simulink model "ADMIRE"  (R2021b)
settings: Solver=ode4  StartTime=0.0  StopTime=100  FixedStep=1e-2  RelTol=1e-3
undefined symbols (not defined in the file or in its folder): admireDB, Earth, WGS84
libraries: simulink_extras x112, simulink x27, aerolibutil x4, dspsigops x4, aerolibfltsims x3, sharedtransform x2, aerolibtransform2 x2, aerolibatmos2 x1, matrix_library x1, sharedutil x1, aerolibanimutils x1, vrlib x1
(part 3 of 15)

== system ADMIRE/Aircraft/Aerodynamics/YawMomentCoefficient/MachRegion2 ==
  note: 0.4 < Mach < 0.5
  AeroIn_Bus : Inport
  Bus Creator : BusCreator  Inputs=3
  Cymbasic : Subsystem
  Cymbcai : Subsystem
  Cymbde : Subsystem
  Cymbdle : Subsystem
  Cymbdn : Subsystem
  Cymbeta : Subsystem
  Cymbetad : Subsystem
  Cymblg : Subsystem
  Cymdai : Subsystem
  Cymdaib : Subsystem
  Cymday : Subsystem
  Cymdayb : Subsystem
  Cymdna : Subsystem
  Cymdr : Subsystem
  Cymp : Subsystem
  Cympbeta : Subsystem
  Cymr : Subsystem
  Cymrbeta : Subsystem
  Sum : Sum  Inputs=18
  eoeff : Subsystem
  Cymtot : Outport
  wires:
  Cympbeta/1(Cympbeta) -> Sum/16  "Cympbeta"
  eoeff/2(eieff) -> Bus Creator/3  "eieff"
  Cymdaib/1(Cymdaib) -> Sum/10  "Cymdaib"
  Cymbdle/1(Cymbdle) -> Sum/5  "Cymbdle"
  Cymdr/1(Cymdr) -> Sum/8  "Cymdr"
  Cymr/1(Cymr) -> Sum/17  "Cymr"
  Cymdayb/1(Cymdayb) -> Sum/12  "Cymdayb"
  Cymdai/1(Cymdai) -> Sum/9  "Cymdai"
  Cymrbeta/1(Cymrbeta) -> Sum/18  "Cymrbeta"
  Bus Creator/1 -> Cympbeta/1(in_bus), Cymr/1(in_bus), Cymrbeta/1(in_bus), Cymp/1(in_bus), Cymbetad/1(in_bus), Cymdna/1(in_bus), Cymdayb/1(in_bus), Cymday/1(in_bus), Cymdaib/1(in_bus), Cymdai/1(in_bus), Cymdr/1(in_bus), Cymblg/1(in_bus), Cymbcai/1(in_bus), Cymbdle/1(in_bus), Cymbdn/1(in_bus), Cymbde/1(in_bus), Cymbeta/1(in_bus), Cymbasic/1(in_bus)  "in_bus"
  eoeff/1(eoeff) -> Bus Creator/2  "eoeff"
  Cymbasic/1(Cymbasic) -> Sum/1  "Cymbasic"
  Cymblg/1(Cymblg) -> Sum/7  "Cymblg"
  Cymbde/1(Cymbde) -> Sum/3  "Cymbde"
  AeroIn_Bus/1 -> eoeff/1(AeroIn_Bus), Bus Creator/1
  Cymbcai/1(Cymbcai) -> Sum/6  "Cymbcai"
  Cymbeta/1(Cymbeta) -> Sum/2  "Cymbeta"
  Cymbdn/1(Cymbdn) -> Sum/4  "Cymbdn"
  Cymp/1(Cymp) -> Sum/15  "Cymp"
  Cymbetad/1(Cymbetad) -> Sum/14  "Cymbetad"
  Cymday/1(Cymday) -> Sum/11  "Cymday"
  Cymdna/1(Cymdna) -> Sum/13  "Cymdna"
  Sum/1 -> Cymtot/1

== system ADMIRE/Aircraft/Aerodynamics/YawMomentCoefficient/MachRegion3 ==
  note: 0.5 <= Mach <= 1.4
  AeroIn_Bus : Inport
  Bus Creator : BusCreator  Inputs=3
  Cymbasic : Subsystem
  Cymbcai : Subsystem
  Cymbde : Subsystem
  Cymbdle : Subsystem
  Cymbdn : Subsystem
  Cymbeta : Subsystem
  Cymbetad : Subsystem
  Cymblg : Subsystem
  Cymdai : Subsystem
  Cymdaib : Subsystem
  Cymday : Subsystem
  Cymdayb : Subsystem
  Cymdna : Subsystem
  Cymdr : Subsystem
  Cymp : Subsystem
  Cympbeta : Subsystem
  Cymr : Subsystem
  Cymrbeta : Subsystem
  Sum : Sum  Inputs=18
  eoeff : Subsystem
  Cymtot : Outport
  wires:
  Cymbasic/1(Cymbasic) -> Sum/1  "Cymbasic"
  Cymp/1(Cymp) -> Sum/15  "Cymp"
  Cymday/1(Cymday) -> Sum/11  "Cymday"
  AeroIn_Bus/1 -> eoeff/1(AeroIn_Bus), Bus Creator/1
  Cympbeta/1(Cympbeta) -> Sum/16  "Cympbeta"
  Cymbde/1(Cymbde) -> Sum/3  "Cymbde"
  Cymdna/1(Cymdna) -> Sum/13  "Cymdna"
  Cymbdn/1(Cymbdn) -> Sum/4  "Cymbdn"
  Bus Creator/1 -> Cymr/1(in_bus), Cymp/1(in_bus), Cymbetad/1(in_bus), Cymdna/1(in_bus), Cymday/1(in_bus), Cymdai/1(in_bus), Cymdr/1(in_bus), Cymblg/1(in_bus), Cymbcai/1(in_bus), Cymbdle/1(in_bus), Cymbdn/1(in_bus), Cymbde/1(in_bus), Cymbeta/1(in_bus)  "in_bus"
  eoeff/2(eieff) -> Bus Creator/3  "eieff"
  Cymdaib/1(Cymdaib) -> Sum/10  "Cymdaib"
  Cymblg/1(Cymblg) -> Sum/7  "Cymblg"
  eoeff/1(eoeff) -> Bus Creator/2  "eoeff"
  Cymdayb/1(Cymdayb) -> Sum/12  "Cymdayb"
  Cymbdle/1(Cymbdle) -> Sum/5  "Cymbdle"
  Cymdr/1(Cymdr) -> Sum/8  "Cymdr"
  Cymdai/1(Cymdai) -> Sum/9  "Cymdai"
  Cymr/1(Cymr) -> Sum/17  "Cymr"
  Cymbetad/1(Cymbetad) -> Sum/14  "Cymbetad"
  Cymbcai/1(Cymbcai) -> Sum/6  "Cymbcai"
  Cymrbeta/1(Cymrbeta) -> Sum/18  "Cymrbeta"
  Cymbeta/1(Cymbeta) -> Sum/2  "Cymbeta"
  Sum/1 -> Cymtot/1

== system ADMIRE/Aircraft/Aerodynamics/YawMomentCoefficient/MachRegion4 ==
  note: 1.4 < Mach
  AeroIn_Bus : Inport
  Bus Creator : BusCreator  Inputs=3
  Cymbasic : Subsystem
  Cymbcai : Subsystem
  Cymbde : Subsystem
  Cymbdle : Subsystem
  Cymbdn : Subsystem
  Cymbeta : Subsystem
  Cymbetad : Subsystem
  Cymblg : Subsystem
  Cymdai : Subsystem
  Cymdaib : Subsystem
  Cymday : Subsystem
  Cymdayb : Subsystem
  Cymdna : Subsystem
  Cymdr : Subsystem
  Cymp : Subsystem
  Cympbeta : Subsystem
  Cymr : Subsystem
  Cymrbeta : Subsystem
  Sum : Sum  Inputs=18
  eoeff : Subsystem
  Cymtot : Outport
  wires:
  Sum/1 -> Cymtot/1
  Cymbeta/1(Cymbeta) -> Sum/2  "Cymbeta"
  Cymrbeta/1(Cymrbeta) -> Sum/18  "Cymrbeta"
  Cymbcai/1(Cymbcai) -> Sum/6  "Cymbcai"
  Cymbetad/1(Cymbetad) -> Sum/14  "Cymbetad"
  Cymr/1(Cymr) -> Sum/17  "Cymr"
  Cymdai/1(Cymdai) -> Sum/9  "Cymdai"
  Cymdr/1(Cymdr) -> Sum/8  "Cymdr"
  Cymbdle/1(Cymbdle) -> Sum/5  "Cymbdle"
  Cymdayb/1(Cymdayb) -> Sum/12  "Cymdayb"
  eoeff/1(eoeff) -> Bus Creator/2  "eoeff"
  Cymblg/1(Cymblg) -> Sum/7  "Cymblg"
  Cymdaib/1(Cymdaib) -> Sum/10  "Cymdaib"
  eoeff/2(eieff) -> Bus Creator/3  "eieff"
  Bus Creator/1 -> Cymbeta/1(in_bus), Cymbde/1(in_bus), Cymbdn/1(in_bus), Cymbdle/1(in_bus), Cymbcai/1(in_bus), Cymblg/1(in_bus), Cymdr/1(in_bus), Cymdai/1(in_bus), Cymday/1(in_bus), Cymdna/1(in_bus), Cymbetad/1(in_bus), Cymp/1(in_bus), Cymr/1(in_bus)  "in_bus"
  Cymbdn/1(Cymbdn) -> Sum/4  "Cymbdn"
  Cymdna/1(Cymdna) -> Sum/13  "Cymdna"
  Cymbde/1(Cymbde) -> Sum/3  "Cymbde"
  Cympbeta/1(Cympbeta) -> Sum/16  "Cympbeta"
  AeroIn_Bus/1 -> Bus Creator/1, eoeff/1(AeroIn_Bus)
  Cymday/1(Cymday) -> Sum/11  "Cymday"
  Cymp/1(Cymp) -> Sum/15  "Cymp"
  Cymbasic/1(Cymbasic) -> Sum/1  "Cymbasic"

== system ADMIRE/Aircraft/Aerodynamics/YawMomentCoefficient/Subsystem ==
  mach_nd : Inport
  CymtotMR1 : Inport  Port=2
  CymtotMR2 : Inport  Port=3
  CymtotMR3 : Inport  Port=4
  CymtotMR4 : Inport  Port=5
  AND : Logic  IconShape=distinctive  AllPortsSameDT=off  OutDataTypeStr=boolean
  AND1 : Logic  IconShape=distinctive  AllPortsSameDT=off  OutDataTypeStr=boolean
  Compare To Constant1 : simulink/Logic and Bit Operations/Compare To Constant  relop=<=  const=0.4  OutDataTypeStr=boolean
  Compare To Constant2 : simulink/Logic and Bit Operations/Compare To Constant  relop=>  const=0.4  OutDataTypeStr=boolean
  Compare To Constant3 : simulink/Logic and Bit Operations/Compare To Constant  relop=<  const=0.5  OutDataTypeStr=boolean
  Compare To Constant4 : simulink/Logic and Bit Operations/Compare To Constant  relop=<=  const=1.4  OutDataTypeStr=boolean
  Compare To Constant5 : simulink/Logic and Bit Operations/Compare To Constant  relop=>=  const=0.5  OutDataTypeStr=boolean
  Switch : Switch  Criteria=u2 ~= 0
  Switch1 : Switch  Criteria=u2 ~= 0
  Switch2 : Switch  Criteria=u2 ~= 0
  Cymtot : Outport
  wires:
  Compare To Constant5/1 -> AND1/1
  Compare To Constant4/1 -> AND1/2
  AND1/1 -> Switch2/2
  CymtotMR4/1 -> Switch2/3
  CymtotMR3/1 -> Switch2/1
  Switch/1 -> Cymtot/1
  Switch2/1 -> Switch1/3
  CymtotMR2/1 -> Switch1/1
  Switch1/1 -> Switch/3
  CymtotMR1/1 -> Switch/1
  AND/1 -> Switch1/2
  Compare To Constant3/1 -> AND/2
  Compare To Constant2/1 -> AND/1
  Compare To Constant1/1 -> Switch/2
  mach_nd/1 -> Compare To Constant1/1, Compare To Constant3/1, Compare To Constant4/1, Compare To Constant5/1, Compare To Constant2/1

== system ADMIRE/Aircraft/ControlSurfaces/Actuator/Directfeed ==
  In Bus Element : Inport  PortName=actIn  Element=outElevonRCmd_deg
  In Bus Element1 : Inport  PortName=actIn  Element=canardRCmd_deg
  In Bus Element2 : Inport  PortName=actIn  Element=rudderCmd_deg
  In Bus Element3 : Inport  PortName=actIn  Element=thrustCmd_pct
  In Bus Element4 : Inport  PortName=actIn  Element=canardLCmd_deg
  In Bus Element5 : Inport  PortName=actIn  Element=outElevonLCmd_deg
  In Bus Element6 : Inport  PortName=actIn  Element=inElevonLCmd_deg
  In Bus Element7 : Inport  PortName=actIn  Element=inElevonRCmd_deg
  In Bus Element8 : Inport  PortName=actIn  Element=lefCmd_deg
  In Bus Element9 : Inport  PortName=actIn  Element=lgCmd_bool
  Out Bus Element : Outport  PortName=actOut  Element=outElevonR_deg
  Out Bus Element1 : Outport  PortName=actOut  Element=canardR_deg
  Out Bus Element2 : Outport  PortName=actOut  Element=rudder_deg
  Out Bus Element3 : Outport  PortName=actOut  Element=thrust_pct
  Out Bus Element4 : Outport  PortName=actOut  Element=canardL_deg
  Out Bus Element5 : Outport  PortName=actOut  Element=outElevonL_deg
  Out Bus Element6 : Outport  PortName=actOut  Element=inElevonL_deg
  Out Bus Element7 : Outport  PortName=actOut  Element=inElevonR_deg
  Out Bus Element8 : Outport  PortName=actOut  Element=lef_deg
  Out Bus Element9 : Outport  PortName=actOut  Element=lg_bool
  wires:
  In Bus Element/1 -> Out Bus Element/1
  In Bus Element1/1 -> Out Bus Element1/1
  In Bus Element2/1 -> Out Bus Element2/1
  In Bus Element3/1 -> Out Bus Element3/1
  In Bus Element4/1 -> Out Bus Element4/1
  In Bus Element5/1 -> Out Bus Element5/1
  In Bus Element6/1 -> Out Bus Element6/1
  In Bus Element7/1 -> Out Bus Element7/1
  In Bus Element8/1 -> Out Bus Element8/1
  In Bus Element9/1 -> Out Bus Element9/1

== system ADMIRE/Aircraft/ControlSurfaces/Actuator/FirstOrder ==
  In Bus Element : Inport  PortName=actIn  Element=outElevonRCmd_deg
  In Bus Element1 : Inport  PortName=actIn  Element=canardRCmd_deg
  In Bus Element2 : Inport  PortName=actIn  Element=rudderCmd_deg
  In Bus Element3 : Inport  PortName=actIn  Element=thrustCmd_pct
  In Bus Element4 : Inport  PortName=actIn  Element=canardLCmd_deg
  In Bus Element5 : Inport  PortName=actIn  Element=outElevonLCmd_deg
  In Bus Element6 : Inport  PortName=actIn  Element=inElevonLCmd_deg
  In Bus Element7 : Inport  PortName=actIn  Element=inElevonRCmd_deg
  In Bus Element8 : Inport  PortName=actIn  Element=lefCmd_deg
  In Bus Element9 : Inport  PortName=actIn  Element=lgCmd_bool
  canardL : Subsystem
  inElevonL : Subsystem
  inElevonR : Subsystem
  lef : Subsystem
  outCanardR : Subsystem
  outElevonL : Subsystem
  outElevonR : Subsystem
  rudder : Subsystem
  Out Bus Element : Outport  PortName=actOut  Element=outElevonR_deg
  Out Bus Element1 : Outport  PortName=actOut  Element=canardR_deg
  Out Bus Element2 : Outport  PortName=actOut  Element=rudder_deg
  Out Bus Element3 : Outport  PortName=actOut  Element=thrust_pct
  Out Bus Element4 : Outport  PortName=actOut  Element=canardL_deg
  Out Bus Element5 : Outport  PortName=actOut  Element=outElevonL_deg
  Out Bus Element6 : Outport  PortName=actOut  Element=inElevonL_deg
  Out Bus Element7 : Outport  PortName=actOut  Element=inElevonR_deg
  Out Bus Element8 : Outport  PortName=actOut  Element=lef_deg
  Out Bus Element9 : Outport  PortName=actOut  Element=lg_bool
  wires:
  In Bus Element/1 -> outElevonR/1(actIn)
  In Bus Element1/1 -> outCanardR/1(actIn)
  In Bus Element2/1 -> rudder/1(actIn)
  In Bus Element4/1 -> canardL/1(actIn)
  In Bus Element5/1 -> outElevonL/1(actIn)
  In Bus Element6/1 -> inElevonL/1(actIn)
  In Bus Element7/1 -> inElevonR/1(actIn)
  In Bus Element8/1 -> lef/1(actIn)
  outElevonR/1(actOut) -> Out Bus Element/1
  outCanardR/1(actOut) -> Out Bus Element1/1
  In Bus Element9/1 -> Out Bus Element9/1
  lef/1(actOut) -> Out Bus Element8/1
  inElevonR/1(actOut) -> Out Bus Element7/1
  inElevonL/1(actOut) -> Out Bus Element6/1
  outElevonL/1(actOut) -> Out Bus Element5/1
  canardL/1(actOut) -> Out Bus Element4/1
  In Bus Element3/1 -> Out Bus Element3/1
  rudder/1(actOut) -> Out Bus Element2/1

== system ADMIRE/Aircraft/Equtions of Motion/Angular Speeds/Subsystem ==
  In1 : Inport
  Bus Selector : BusSelector  OutputSignals=Aero_Bus.aeroMomentBodyX_N,Aero_Bus.aeroMomentBodyY_N,Aero_Bus.aeroMomentBodyZ_N
  Ground : Ground
  Mux : Mux  Inputs=3
  Mux1 : Mux  Inputs=3
  Mux2 : Mux  Inputs=3
  Sum : Sum  Inputs=+++
  Out1 : Outport
  wires:
  In1/1 -> Bus Selector/1
  Bus Selector/1 -> Mux/1  "<aeroMomentBodyX_N>"
  Bus Selector/2 -> Mux/2  "<aeroMomentBodyY_N>"
  Bus Selector/3 -> Mux/3  "<aeroMomentBodyZ_N>"
  Mux1/1 -> Sum/2
  Mux/1 -> Sum/1
  Mux2/1 -> Sum/3
  Sum/1 -> Out1/1
  Ground/1 -> Mux2/3, Mux2/2, Mux2/1, Mux1/3, Mux1/2, Mux1/1

== system ADMIRE/Aircraft/Equtions of Motion/Translational Speeds/Angle of Attack Equation ==
  ForcesWindAxes : Inport
  Flow : Inport  Port=2
  Bus Selector : BusSelector  OutputSignals=Mass_Bus.mass_kg,EOM_Bus.speedWindX_mps,EOM_Bus.angleOfAttack_rad,EOM_Bus.angleOfSideslip_rad,EOM_Bus.angularSpeedBodyX_rps,EOM_Bus.angularSpeedBodyY_rps,EOM_Bus.angularSpeedBodyZ_rps
  Constant : Constant
  Cos : Trigonometry  Operator=cos
  Cos1 : Trigonometry  Operator=cos
  Cos2 : Trigonometry
  Cos3 : Trigonometry  Operator=tan
  Max : MinMax  Function=max  Inputs=2
  Product : Product  Inputs=*///
  Product1 : Product
  Product2 : Product
  Product3 : Product
  Selector : Selector  InputPortWidth=3  IndexOptions=Index vector (dialog)  Indices=3  OutputSizes=1
  Sum1 : Sum  Inputs=|++
  Sum2 : Sum  Inputs=++-
  angleOfAttack_rad : Integrator  ContinuousStateAttributes='angleOfAttack_rad'
  aoa : Outport
  aoaDot : Outport  Port=2
  wires:
  Bus Selector/1 -> [m]  "<mass_kg>"
  Flow/1 -> Bus Selector/1
  Selector/1 -> Product/1
  Bus Selector/2 -> [vt]  "<speedWindX_mps>"
  [aos] -> Cos/1
  Cos/1 -> Product/3
  [m] -> Product/2
  [aoa] -> Cos2/1, Cos1/1
  Cos1/1 -> Product1/2
  [p] -> Product1/1
  [r] -> Product2/1
  Cos2/1 -> Product2/2
  Product1/1 -> Sum1/1
  Product2/1 -> Sum1/2
  Sum1/1 -> Product3/1
  Cos3/1 -> Product3/2
  [aos] -> Cos3/1
  [q] -> Sum2/2
  Product/1 -> Sum2/1
  Product3/1 -> Sum2/3
  Sum2/1 -> aoaDot/1, angleOfAttack_rad/1
  angleOfAttack_rad/1 -> aoa/1  "angleOfAttack_rad"
  Bus Selector/3 -> [aoa]  "<angleOfAttack_rad>"
  Bus Selector/4 -> [aos]  "<angleOfSideslip_rad>"
  Bus Selector/5 -> [p]  "<angularSpeedBodyX_rps>"
  Bus Selector/7 -> [r]  "<angularSpeedBodyZ_rps>"
  [vt] -> Max/1
  Max/1 -> Product/4
  Constant/1 -> Max/2
  Bus Selector/6 -> [q]  "<angularSpeedBodyY_rps>"
  ForcesWindAxes/1 -> Selector/1

== system ADMIRE/Aircraft/Equtions of Motion/Translational Speeds/Angle of Sideslip Equation ==
  ForcesWindAxes : Inport
  Flow : Inport  Port=2
  Bus Selector : BusSelector  OutputSignals=Mass_Bus.mass_kg,EOM_Bus.speedWindX_mps,EOM_Bus.angleOfAttack_rad,EOM_Bus.angularSpeedBodyX_rps,EOM_Bus.angularSpeedBodyZ_rps
  Constant : Constant
  Cos : Trigonometry  Operator=cos
  Cos1 : Trigonometry
  Max : MinMax  Function=max  Inputs=2
  Product : Product  Inputs=*//
  Product1 : Product
  Product2 : Product
  Selector : Selector  InputPortWidth=3  IndexOptions=Index vector (dialog)  Indices=2  OutputSizes=1
  Sum2 : Sum  Inputs=++-
  angleOfSideslip_rad : Integrator  ContinuousStateAttributes='angleOfSideslip_rad'
  aos : Outport
  aosDot : Outport  Port=2
  wires:
  Flow/1 -> Bus Selector/1
  [aoa] -> Cos/1, Cos1/1
  Cos1/1 -> Product1/2
  [p] -> Product1/1
  [r] -> Product2/1
  Cos/1 -> Product2/2
  Product1/1 -> Sum2/2
  Product2/1 -> Sum2/3
  Product/1 -> Sum2/1
  angleOfSideslip_rad/1 -> aos/1  "angleOfSideslip_rad"
  Sum2/1 -> aosDot/1, angleOfSideslip_rad/1
  Bus Selector/2 -> [vt]  "<speedWindX_mps>"
  Bus Selector/1 -> [m]  "<mass_kg>"
  Bus Selector/3 -> [aoa]  "<angleOfAttack_rad>"
  Bus Selector/4 -> [p]  "<angularSpeedBodyX_rps>"
  Bus Selector/5 -> [r]  "<angularSpeedBodyZ_rps>"
  [m] -> Product/2
  [vt] -> Max/1
  Max/1 -> Product/3
  Constant/1 -> Max/2
  ForcesWindAxes/1 -> Selector/1
  Selector/1 -> Product/1

== system ADMIRE/Aircraft/Equtions of Motion/Translational Speeds/ForcesWindAxes ==
  Flow : Inport
  Bus Selector1 : BusSelector  OutputSignals=DCM_Bus.dcmBody2Wind,Mass_Bus.gravForceBodyX_N,Mass_Bus.gravForceBodyY_N,Mass_Bus.gravForceBodyZ_N,Engine_Bus.thrustX_N,Engine_Bus.thrustY_N,Engine_Bus.thrustZ_N,Aero_Bus.aeroForceBodyX_N,Aero_Bus.aeroForceBodyY_N,Aero_Bus.aeroForceBodyZ_N
  Matrix Multiply : Product  Multiplication=Matrix(*)
  Mux : Mux  Inputs=3
  Mux1 : Mux  Inputs=3
  Mux2 : Mux  Inputs=3
  Sum : Sum  Inputs=+++
  ForcesWindAxes : Outport
  wires:
  Flow/1 -> Bus Selector1/1
  Bus Selector1/4 -> Mux/3  "<gravForceBodyZ_N>"
  Bus Selector1/3 -> Mux/2  "<gravForceBodyY_N>"
  Bus Selector1/2 -> Mux/1  "<gravForceBodyX_N>"
  Bus Selector1/6 -> Mux1/2  "<thrustY_N>"
  Bus Selector1/7 -> Mux1/3  "<thrustZ_N>"
  Bus Selector1/5 -> Mux1/1  "<thrustX_N>"
  Bus Selector1/8 -> Mux2/1  "<aeroForceBodyX_N>"
  Bus Selector1/9 -> Mux2/2  "<aeroForceBodyY_N>"
  Bus Selector1/10 -> Mux2/3  "<aeroForceBodyZ_N>"
  Mux1/1 -> Sum/2
  Mux/1 -> Sum/1
  Mux2/1 -> Sum/3
  Bus Selector1/1 -> Matrix Multiply/1  "<dcmBody2Wind>"
  Sum/1 -> Matrix Multiply/2
  Matrix Multiply/1 -> ForcesWindAxes/1

== system ADMIRE/Aircraft/Equtions of Motion/Translational Speeds/V Equation ==
  ForcesWindAxes : Inport
  Flow : Inport  Port=2
  Bus Selector : BusSelector  OutputSignals=Mass_Bus.mass_kg
  Product1 : Product  Inputs=*/
  Selector : Selector  InputPortWidth=3  IndexOptions=Index vector (dialog)  Indices=1  OutputSizes=1
  speedWindX_mps : Integrator  ContinuousStateAttributes='speedWindX_mps'
  V : Outport
  VDot : Outport  Port=2
  wires:
  Flow/1 -> Bus Selector/1
  Bus Selector/1 -> Product1/2  "<mass_kg>"
  ForcesWindAxes/1 -> Selector/1
  Product1/1 -> speedWindX_mps/1, VDot/1
  speedWindX_mps/1 -> V/1  "speedWindX_mps"
  Selector/1 -> Product1/1

== system ADMIRE/Aircraft/Aerodynamics/CentripetalForceCoefficient/MachRegion1/Ccbcai ==
  in_bus : Inport
  Bus Selector : BusSelector  OutputSignals=AeroIn_Bus.cai,AeroIn_Bus.angleOfAttack_deg,AeroIn_Bus.angleOfSideslip_deg
  Ccbcai_ : Subsystem
  Ccbcai : Outport
  wires:
  Bus Selector/3 -> Ccbcai_/3(angleOfSideslip_deg)  "<angleOfSideslip_deg>"
  Bus Selector/2 -> Ccbcai_/2(angleOfAttack_deg)  "<angleOfAttack_deg>"
  in_bus/1 -> Bus Selector/1  "in_bus"
  Ccbcai_/1(Ccbcai) -> Ccbcai/1
  Bus Selector/1 -> Ccbcai_/1(CAI)  "<cai>"

== system ADMIRE/Aircraft/Aerodynamics/CentripetalForceCoefficient/MachRegion1/Ccbde ==
  in_bus : Inport
  Bus Selector : BusSelector  OutputSignals=AeroIn_Bus.angleOfSideslip_deg,AeroIn_Bus.dEI,AeroIn_Bus.angleOfAttack_deg,eieff,AeroIn_Bus.dEY,eoeff
  Ccbde_ : Subsystem
  Ccbde : Outport
  wires:
  Bus Selector/6 -> Ccbde_/6(eoeff)  "<eoeff>"
  Bus Selector/5 -> Ccbde_/5(dEY)  "<dEY>"
  Bus Selector/4 -> Ccbde_/4(eieff)  "<eieff>"
  Bus Selector/3 -> Ccbde_/3(angleOfAttack_deg)  "<angleOfAttack_deg>"
  Bus Selector/2 -> Ccbde_/2(dEI)  "<dEI>"
  Bus Selector/1 -> Ccbde_/1(angleOfSideslip_deg)  "<angleOfSideslip_deg>"
  Ccbde_/1(Ccbde) -> Ccbde/1
  in_bus/1 -> Bus Selector/1  "in_bus"

== system ADMIRE/Aircraft/Aerodynamics/CentripetalForceCoefficient/MachRegion1/Ccbdle ==
  in_bus : Inport
  Bus Selector : BusSelector  OutputSignals=AeroIn_Bus.lef_deg,AeroIn_Bus.angleOfSideslip_deg,AeroIn_Bus.angleOfAttack_deg
  Ccbdle_ : Subsystem
  Ccbdle : Outport
  wires:
  Bus Selector/3 -> Ccbdle_/3(angleOfAttack_deg)  "<angleOfAttack_deg>"
  Bus Selector/2 -> Ccbdle_/2(angleOfSideslip_deg)  "<angleOfSideslip_deg>"
  Bus Selector/1 -> Ccbdle_/1(dLE)  "<lef_deg>"
  Ccbdle_/1(Ccbdle) -> Ccbdle/1
  in_bus/1 -> Bus Selector/1  "in_bus"

== system ADMIRE/Aircraft/Aerodynamics/CentripetalForceCoefficient/MachRegion1/Ccbdn ==
  in_bus : Inport
  Bus Selector : BusSelector  OutputSignals=AeroIn_Bus.angleOfSideslip_deg,AeroIn_Bus.dN,AeroIn_Bus.angleOfAttack_deg
  Ccbdn_ : Subsystem
  Ccbdn : Outport
  wires:
  Bus Selector/2 -> Ccbdn_/2(dN)  "<dN>"
  Bus Selector/1 -> Ccbdn_/1(angleOfSideslip_deg)  "<angleOfSideslip_deg>"
  Bus Selector/3 -> Ccbdn_/3(angleOfAttack_deg)  "<angleOfAttack_deg>"
  in_bus/1 -> Bus Selector/1  "in_bus"
  Ccbdn_/1(Ccbdn) -> Ccbdn/1

== system ADMIRE/Aircraft/Aerodynamics/CentripetalForceCoefficient/MachRegion1/Ccbeta ==
  in_bus : Inport
  Bus Selector : BusSelector  OutputSignals=AeroIn_Bus.angleOfSideslip_deg,AeroIn_Bus.angleOfAttack_deg,AeroIn_Bus.qacorr,AeroIn_Bus.mach_nd
  Ccbeta_ : Subsystem
  Ccbeta : Outport
  wires:
  Ccbeta_/1(Ccbeta) -> Ccbeta/1
  Bus Selector/4 -> Ccbeta_/4(mach_nd)  "<mach_nd>"
  Bus Selector/3 -> Ccbeta_/3(qacorr)  "<qacorr>"
  Bus Selector/2 -> Ccbeta_/2(angleOfAttack_deg)  "<angleOfAttack_deg>"
  Bus Selector/1 -> Ccbeta_/1(angleOfSideslip_deg)  "<angleOfSideslip_deg>"
  in_bus/1 -> Bus Selector/1  "in_bus"

== system ADMIRE/Aircraft/Aerodynamics/CentripetalForceCoefficient/MachRegion1/Ccbetad ==
  in_bus : Inport
  Bus Selector : BusSelector  OutputSignals=AeroIn_Bus.angleOfAttack_deg,AeroIn_Bus.betad
  Ccbetad_ : Subsystem
  Ccbetad : Outport
  wires:
  Bus Selector/2 -> Ccbetad_/2(betad)  "<betad>"
  Bus Selector/1 -> Ccbetad_/1(angleOfAttack_deg)  "<angleOfAttack_deg>"
  in_bus/1 -> Bus Selector/1  "in_bus"
  Ccbetad_/1(Ccbetad) -> Ccbetad/1

== system ADMIRE/Aircraft/Aerodynamics/CentripetalForceCoefficient/MachRegion1/Ccblg ==
  in_bus : Inport
  Bus Selector : BusSelector  OutputSignals=AeroIn_Bus.lg_bool,AeroIn_Bus.angleOfAttack_deg,AeroIn_Bus.angleOfSideslip_deg
  Ccblg_ : Subsystem
  Ccblg : Outport
  wires:
  Bus Selector/1 -> Ccblg_/1(dLG)  "<lg_bool>"
  Bus Selector/3 -> Ccblg_/3(angleOfSideslip_deg)  "<angleOfSideslip_deg>"
  Bus Selector/2 -> Ccblg_/2(angleOfAttack_deg)  "<angleOfAttack_deg>"
  in_bus/1 -> Bus Selector/1  "in_bus"
  Ccblg_/1(Ccblg) -> Ccblg/1

== system ADMIRE/Aircraft/Aerodynamics/CentripetalForceCoefficient/MachRegion1/Ccdai ==
  in_bus : Inport
  Bus Selector : BusSelector  OutputSignals=AeroIn_Bus.dAI,AeroIn_Bus.angleOfAttack_deg,AeroIn_Bus.dEI,eieff,AeroIn_Bus.qacorr,AeroIn_Bus.mach_nd
  Ccdai_ : Subsystem
  Ccdai : Outport
  wires:
  Bus Selector/1 -> Ccdai_/1(dAI)  "<dAI>"
  Bus Selector/2 -> Ccdai_/2(angleOfAttack_deg)  "<angleOfAttack_deg>"
  Bus Selector/3 -> Ccdai_/3(dEI)  "<dEI>"
  Bus Selector/4 -> Ccdai_/4(eieff)  "<eieff>"
  Bus Selector/5 -> Ccdai_/5(qacorr)  "<qacorr>"
  Bus Selector/6 -> Ccdai_/6(mach_nd)  "<mach_nd>"
  in_bus/1 -> Bus Selector/1  "in_bus"
  Ccdai_/1(Ccdai) -> Ccdai/1

== system ADMIRE/Aircraft/Aerodynamics/CentripetalForceCoefficient/MachRegion1/Ccdaib ==
  in_bus : Inport
  Bus Selector : BusSelector  OutputSignals=AeroIn_Bus.angleOfAttack_deg,AeroIn_Bus.dAI,AeroIn_Bus.angleOfSideslip_deg,eieff
  Ccdaib_ : Subsystem
  Ccdaib : Outport
  wires:
  Bus Selector/4 -> Ccdaib_/4(eieff)  "<eieff>"
  Bus Selector/3 -> Ccdaib_/3(angleOfSideslip_deg)  "<angleOfSideslip_deg>"
  Bus Selector/1 -> Ccdaib_/1(angleOfAttack_deg)  "<angleOfAttack_deg>"
  Bus Selector/2 -> Ccdaib_/2(dAI)  "<dAI>"
  Ccdaib_/1(Ccdaib) -> Ccdaib/1
  in_bus/1 -> Bus Selector/1  "in_bus"

== system ADMIRE/Aircraft/Aerodynamics/CentripetalForceCoefficient/MachRegion1/Ccday ==
  in_bus : Inport
  Bus Selector : BusSelector  OutputSignals=AeroIn_Bus.dAY,AeroIn_Bus.angleOfAttack_deg,AeroIn_Bus.dEY,eoeff,AeroIn_Bus.qacorr,AeroIn_Bus.mach_nd
  Ccday_ : Subsystem
  Ccday : Outport
  wires:
  Ccday_/1(Ccday) -> Ccday/1
  in_bus/1 -> Bus Selector/1  "in_bus"
  Bus Selector/6 -> Ccday_/6(mach_nd)  "<mach_nd>"
  Bus Selector/5 -> Ccday_/5(qacorr)  "<qacorr>"
  Bus Selector/4 -> Ccday_/4(eoeff)  "<eoeff>"
  Bus Selector/3 -> Ccday_/3(dEY)  "<dEY>"
  Bus Selector/2 -> Ccday_/2(angleOfAttack_deg)  "<angleOfAttack_deg>"
  Bus Selector/1 -> Ccday_/1(dAY)  "<dAY>"

== system ADMIRE/Aircraft/Aerodynamics/CentripetalForceCoefficient/MachRegion1/Ccdayb ==
  in_bus : Inport
  Bus Selector : BusSelector  OutputSignals=AeroIn_Bus.angleOfAttack_deg,AeroIn_Bus.dAY,AeroIn_Bus.angleOfSideslip_deg,eoeff
  Ccdayb_ : Subsystem
  Ccdayb : Outport
  wires:
  in_bus/1 -> Bus Selector/1  "in_bus"
  Ccdayb_/1(Ccdayb) -> Ccdayb/1
  Bus Selector/2 -> Ccdayb_/2(dAY)  "<dAY>"
  Bus Selector/1 -> Ccdayb_/1(angleOfAttack_deg)  "<angleOfAttack_deg>"
  Bus Selector/3 -> Ccdayb_/3(angleOfSideslip_deg)  "<angleOfSideslip_deg>"
  Bus Selector/4 -> Ccdayb_/4(eoeff)  "<eoeff>"

== system ADMIRE/Aircraft/Aerodynamics/CentripetalForceCoefficient/MachRegion1/Ccdna ==
  in_bus : Inport
  Bus Selector : BusSelector  OutputSignals=AeroIn_Bus.dNE,AeroIn_Bus.angleOfAttack_deg,AeroIn_Bus.dNA
  Ccdna_ : Subsystem
  Ccdna : Outport
  wires:
  Bus Selector/3 -> Ccdna_/3(dNA)  "<dNA>"
  Bus Selector/1 -> Ccdna_/1(dNE)  "<dNE>"
  Bus Selector/2 -> Ccdna_/2(angleOfAttack_deg)  "<angleOfAttack_deg>"
  Ccdna_/1(Ccdna) -> Ccdna/1
  in_bus/1 -> Bus Selector/1  "in_bus"

== system ADMIRE/Aircraft/Aerodynamics/CentripetalForceCoefficient/MachRegion1/Ccdr ==
  in_bus : Inport
  Bus Selector : BusSelector  OutputSignals=AeroIn_Bus.angleOfAttack_deg,AeroIn_Bus.rud_deg,AeroIn_Bus.angleOfSideslip_deg,AeroIn_Bus.qacorr,AeroIn_Bus.mach_nd
  Ccdr_ : Subsystem
  Ccdr : Outport
  wires:
  Ccdr_/1(Ccdr) -> Ccdr/1
  Bus Selector/1 -> Ccdr_/1(angleOfAttack_deg)  "<angleOfAttack_deg>"
  Bus Selector/2 -> Ccdr_/2(dR)  "<rud_deg>"
  Bus Selector/3 -> Ccdr_/3(angleOfSideslip_deg)  "<angleOfSideslip_deg>"
  Bus Selector/4 -> Ccdr_/4(qacorr)  "<qacorr>"
  Bus Selector/5 -> Ccdr_/5(mach_nd)  "<mach_nd>"
  in_bus/1 -> Bus Selector/1  "in_bus"

== system ADMIRE/Aircraft/Aerodynamics/CentripetalForceCoefficient/MachRegion1/Ccp ==
  in_bus : Inport
  Bus Selector : BusSelector  OutputSignals=AeroIn_Bus.angleOfAttack_deg,AeroIn_Bus.pc
  Ccp_ : Subsystem
  Ccp : Outport
  wires:
  Ccp_/1(Ccp) -> Ccp/1
  in_bus/1 -> Bus Selector/1  "in_bus"
  Bus Selector/1 -> Ccp_/1(angleOfAttack_deg)  "<angleOfAttack_deg>"
  Bus Selector/2 -> Ccp_/2(pc)  "<pc>"

== system ADMIRE/Aircraft/Aerodynamics/CentripetalForceCoefficient/MachRegion1/Ccpbeta ==
  in_bus : Inport
  Bus Selector : BusSelector  OutputSignals=AeroIn_Bus.angleOfSideslip_deg,AeroIn_Bus.pc,AeroIn_Bus.angleOfAttack_deg
  Ccpbeta_ : Subsystem
  Ccpbeta : Outport
  wires:
  Bus Selector/3 -> Ccpbeta_/3(angleOfAttack_deg)  "<angleOfAttack_deg>"
  Bus Selector/1 -> Ccpbeta_/1(angleOfSideslip_deg)  "<angleOfSideslip_deg>"
  Bus Selector/2 -> Ccpbeta_/2(pc)  "<pc>"
  in_bus/1 -> Bus Selector/1  "in_bus"
  Ccpbeta_/1(Ccpbeta) -> Ccpbeta/1

== system ADMIRE/Aircraft/Aerodynamics/CentripetalForceCoefficient/MachRegion1/Ccr ==
  in_bus : Inport
  Bus Selector : BusSelector  OutputSignals=AeroIn_Bus.dN,AeroIn_Bus.angleOfAttack_deg,AeroIn_Bus.rc
  Ccr_ : Subsystem
  Ccr : Outport
  wires:
  Bus Selector/1 -> Ccr_/1(dN)  "<dN>"
  Bus Selector/3 -> Ccr_/3(rc)  "<rc>"
  Bus Selector/2 -> Ccr_/2(angleOfAttack_deg)  "<angleOfAttack_deg>"
  Ccr_/1(Ccr) -> Ccr/1
  in_bus/1 -> Bus Selector/1  "in_bus"

== system ADMIRE/Aircraft/Aerodynamics/CentripetalForceCoefficient/MachRegion1/Ccrbeta ==
  in_bus : Inport
  Bus Selector : BusSelector  OutputSignals=AeroIn_Bus.angleOfSideslip_deg,AeroIn_Bus.angleOfAttack_deg,AeroIn_Bus.rc
  Ccrbeta_ : Subsystem
  Ccrbeta : Outport
  wires:
  Bus Selector/3 -> Ccrbeta_/3(rc)  "<rc>"
  Bus Selector/1 -> Ccrbeta_/1(angleOfSideslip_deg)  "<angleOfSideslip_deg>"
  Bus Selector/2 -> Ccrbeta_/2(angleOfAttack_deg)  "<angleOfAttack_deg>"
  in_bus/1 -> Bus Selector/1  "in_bus"
  Ccrbeta_/1(Ccrbeta) -> Ccrbeta/1

== system ADMIRE/Aircraft/Aerodynamics/CentripetalForceCoefficient/MachRegion1/eoeff1 ==
  AeroIn_Bus : Inport
  Bus Selector : BusSelector  OutputSignals=mach_nd
  CCDAYOD_M : Lookup_n-D  NumberOfTableDimensions=1  BreakpointsForDimension1=admireDB.aerodata_asym_ext.CCDAYOD.breakpoints.M  BreakpointsForDimension3=[5, 7]  Table=admireDB.aerodata_asym_ext.CCDAYOD.newTable  ExtrapMethod=Clip  InternalRulePriority=Speed  RndMeth=Simplest  InputSameDT=on
  Constant : Constant
  Sum : Sum  Inputs=-+|
  eoeff : Outport
  eieff : Outport  Port=2
  wires:
  Sum/1 -> eieff/1
  CCDAYOD_M/1 -> eoeff/1, Sum/1
  Constant/1 -> Sum/2
  Bus Selector/1 -> CCDAYOD_M/1  "<mach_nd>"
  AeroIn_Bus/1 -> Bus Selector/1

== system ADMIRE/Aircraft/Aerodynamics/CentripetalForceCoefficient/MachRegion2/Ccbcai ==
  in_bus : Inport
  Bus Selector : BusSelector  OutputSignals=AeroIn_Bus.cai,AeroIn_Bus.angleOfAttack_deg,AeroIn_Bus.angleOfSideslip_deg
  Ccbcai_ : Subsystem
  Ccbcai : Outport
  wires:
  Bus Selector/1 -> Ccbcai_/1(cai)  "<cai>"
  Bus Selector/3 -> Ccbcai_/3(angleOfSideslip_deg)  "<angleOfSideslip_deg>"
  Bus Selector/2 -> Ccbcai_/2(angleOfAttack_deg)  "<angleOfAttack_deg>"
  in_bus/1 -> Bus Selector/1  "in_bus"
  Ccbcai_/1(Ccbcai) -> Ccbcai/1

== system ADMIRE/Aircraft/Aerodynamics/CentripetalForceCoefficient/MachRegion2/Ccbde ==
  in_bus : Inport
  Bus Selector : BusSelector  OutputSignals=AeroIn_Bus.angleOfAttack_deg,AeroIn_Bus.dEI,AeroIn_Bus.angleOfSideslip_deg,eieff,AeroIn_Bus.dEY,eoeff
  Ccbde_ : Subsystem
  Ccbde : Outport
  wires:
  Bus Selector/1 -> Ccbde_/1(angleOfAttack_deg)  "<angleOfAttack_deg>"
  Bus Selector/2 -> Ccbde_/2(dEI)  "<dEI>"
  Bus Selector/3 -> Ccbde_/3(angleOfSideslip_deg)  "<angleOfSideslip_deg>"
  Bus Selector/4 -> Ccbde_/4(eieff)  "<eieff>"
  Bus Selector/5 -> Ccbde_/5(dEY)  "<dEY>"
  Bus Selector/6 -> Ccbde_/6(eoeff)  "<eoeff>"
  Ccbde_/1(Ccbde) -> Ccbde/1
  in_bus/1 -> Bus Selector/1  "in_bus"

== system ADMIRE/Aircraft/Aerodynamics/CentripetalForceCoefficient/MachRegion2/Ccbdle ==
  in_bus : Inport
  Bus Selector : BusSelector  OutputSignals=AeroIn_Bus.angleOfAttack_deg,AeroIn_Bus.angleOfSideslip_deg,AeroIn_Bus.lef_deg,AeroIn_Bus.tflow,AeroIn_Bus.tfhigh
  Ccbdle_ : Subsystem
  Ccbdle : Outport
  wires:
  Bus Selector/5 -> Ccbdle_/5(tfhigh)  "<tfhigh>"
  Bus Selector/4 -> Ccbdle_/4(tflow)  "<tflow>"
  Bus Selector/3 -> Ccbdle_/3(dLE)  "<lef_deg>"
  Bus Selector/2 -> Ccbdle_/2(angleOfSideslip_deg)  "<angleOfSideslip_deg>"
  Bus Selector/1 -> Ccbdle_/1(angleOfAttack_deg)  "<angleOfAttack_deg>"
  Ccbdle_/1(Ccbdle) -> Ccbdle/1
  in_bus/1 -> Bus Selector/1  "in_bus"

== system ADMIRE/Aircraft/Aerodynamics/CentripetalForceCoefficient/MachRegion2/Ccbdn ==
  in_bus : Inport
  Bus Selector : BusSelector  OutputSignals=AeroIn_Bus.angleOfAttack_deg,AeroIn_Bus.dN,AeroIn_Bus.angleOfSideslip_deg
  Ccbdn_ : Subsystem
  Ccbdn : Outport
  wires:
  Bus Selector/1 -> Ccbdn_/1(angleOfAttack_deg)  "<angleOfAttack_deg>"
  Bus Selector/2 -> Ccbdn_/2(dN)  "<dN>"
  Bus Selector/3 -> Ccbdn_/3(angleOfSideslip_deg)  "<angleOfSideslip_deg>"
  in_bus/1 -> Bus Selector/1  "in_bus"
  Ccbdn_/1(Ccbdn) -> Ccbdn/1

== system ADMIRE/Aircraft/Aerodynamics/CentripetalForceCoefficient/MachRegion2/Ccbeta ==
  in_bus : Inport
  Bus Selector : BusSelector  OutputSignals=AeroIn_Bus.angleOfSideslip_deg,AeroIn_Bus.angleOfAttack_deg,AeroIn_Bus.tflow,AeroIn_Bus.tfhigh,AeroIn_Bus.qacorr,AeroIn_Bus.mach_nd
  Ccbeta_ : Subsystem
  Ccbeta : Outport
  wires:
  Bus Selector/6 -> Ccbeta_/6(mach_nd)  "<mach_nd>"
  Bus Selector/5 -> Ccbeta_/5(qacorr)  "<qacorr>"
  Bus Selector/4 -> Ccbeta_/4(tfhigh)  "<tfhigh>"
  Bus Selector/3 -> Ccbeta_/3(tflow)  "<tflow>"
  Bus Selector/2 -> Ccbeta_/2(angleOfAttack_deg)  "<angleOfAttack_deg>"
  Bus Selector/1 -> Ccbeta_/1(angleOfSideslip_deg)  "<angleOfSideslip_deg>"
  Ccbeta_/1(CCbeta) -> Ccbeta/1
  in_bus/1 -> Bus Selector/1  "in_bus"

== system ADMIRE/Aircraft/Aerodynamics/CentripetalForceCoefficient/MachRegion2/Ccbetad ==
  in_bus : Inport
  Bus Selector : BusSelector  OutputSignals=AeroIn_Bus.angleOfAttack_deg,AeroIn_Bus.tflow,AeroIn_Bus.betad,AeroIn_Bus.tfhigh
  CCbetad_ : Subsystem
  Ccbetad : Outport
  wires:
  Bus Selector/4 -> CCbetad_/4(tfhigh)  "<tfhigh>"
  Bus Selector/3 -> CCbetad_/3(betad)  "<betad>"
  Bus Selector/1 -> CCbetad_/1(angleOfAttack_deg)  "<angleOfAttack_deg>"
  Bus Selector/2 -> CCbetad_/2(tflow)  "<tflow>"
  CCbetad_/1(CCbetad) -> Ccbetad/1
  in_bus/1 -> Bus Selector/1  "in_bus"

== system ADMIRE/Aircraft/Aerodynamics/CentripetalForceCoefficient/MachRegion2/Ccblg ==
  in_bus : Inport
  Bus Selector : BusSelector  OutputSignals=AeroIn_Bus.lg_bool,AeroIn_Bus.angleOfAttack_deg,AeroIn_Bus.angleOfSideslip_deg
  Ccblg_ : Subsystem
  Ccblg : Outport
  wires:
  Bus Selector/1 -> Ccblg_/1(ldg)  "<lg_bool>"
  Bus Selector/3 -> Ccblg_/3(angleOfSideslip_deg)  "<angleOfSideslip_deg>"
  Bus Selector/2 -> Ccblg_/2(angleOfAttack_deg)  "<angleOfAttack_deg>"
  in_bus/1 -> Bus Selector/1  "in_bus"
  Ccblg_/1(Ccblg) -> Ccblg/1

== system ADMIRE/Aircraft/Aerodynamics/CentripetalForceCoefficient/MachRegion2/Ccdai ==
  in_bus : Inport
  Bus Selector : BusSelector  OutputSignals=AeroIn_Bus.dAI,AeroIn_Bus.angleOfAttack_deg,AeroIn_Bus.dEI,AeroIn_Bus.qacorr,AeroIn_Bus.mach_nd,AeroIn_Bus.tflow,AeroIn_Bus.tfhigh,eieff
  Ccdai_ : Subsystem
  Ccdai : Outport
  wires:
  Bus Selector/8 -> Ccdai_/8(eieff)  "<eieff>"
  Bus Selector/7 -> Ccdai_/7(tfhigh)  "<tfhigh>"
  Bus Selector/6 -> Ccdai_/6(tflow)  "<tflow>"
  Bus Selector/5 -> Ccdai_/5(mach_nd)  "<mach_nd>"
  Bus Selector/4 -> Ccdai_/4(qacorr)  "<qacorr>"
  Bus Selector/3 -> Ccdai_/3(dEI)  "<dEI>"
  Bus Selector/2 -> Ccdai_/2(angleOfAttack_deg)  "<angleOfAttack_deg>"
  Bus Selector/1 -> Ccdai_/1(dAI)  "<dAI>"
  in_bus/1 -> Bus Selector/1  "in_bus"
  Ccdai_/1(Ccdai) -> Ccdai/1

== system ADMIRE/Aircraft/Aerodynamics/CentripetalForceCoefficient/MachRegion2/Ccdaib ==
  in_bus : Inport
  Bus Selector : BusSelector  OutputSignals=AeroIn_Bus.angleOfAttack_deg,AeroIn_Bus.dAI,AeroIn_Bus.angleOfSideslip_deg,AeroIn_Bus.tflow,eieff
  Ccdaib_ : Subsystem
  Ccdaib : Outport
  wires:
  Bus Selector/5 -> Ccdaib_/5(eieff)  "<eieff>"
  Bus Selector/4 -> Ccdaib_/4(tflow)  "<tflow>"
  Bus Selector/3 -> Ccdaib_/3(angleOfSideslip_deg)  "<angleOfSideslip_deg>"
  Bus Selector/2 -> Ccdaib_/2(dAI)  "<dAI>"
  Bus Selector/1 -> Ccdaib_/1(angleOfAttack_deg)  "<angleOfAttack_deg>"
  Ccdaib_/1(Ccdaib) -> Ccdaib/1
  in_bus/1 -> Bus Selector/1  "in_bus"

== system ADMIRE/Aircraft/Aerodynamics/CentripetalForceCoefficient/MachRegion2/Ccday ==
  in_bus : Inport
  Bus Selector : BusSelector  OutputSignals=AeroIn_Bus.dAY,AeroIn_Bus.angleOfAttack_deg,AeroIn_Bus.dEY,AeroIn_Bus.qacorr,AeroIn_Bus.mach_nd,AeroIn_Bus.tflow,AeroIn_Bus.tfhigh,eoeff
  Ccday_ : Subsystem
  Ccday : Outport
  wires:
  Bus Selector/8 -> Ccday_/8(eoeff)  "<eoeff>"
  Bus Selector/7 -> Ccday_/7(tfhigh)  "<tfhigh>"
  Bus Selector/6 -> Ccday_/6(tflow)  "<tflow>"
  Bus Selector/5 -> Ccday_/5(mach_nd)  "<mach_nd>"
  Bus Selector/4 -> Ccday_/4(qacorr)  "<qacorr>"
  Bus Selector/3 -> Ccday_/3(dEY)  "<dEY>"
  Bus Selector/2 -> Ccday_/2(angleOfAttack_deg)  "<angleOfAttack_deg>"
  Bus Selector/1 -> Ccday_/1(dAY)  "<dAY>"
  in_bus/1 -> Bus Selector/1  "in_bus"
  Ccday_/1(Ccday) -> Ccday/1

== system ADMIRE/Aircraft/Aerodynamics/CentripetalForceCoefficient/MachRegion2/Ccdayb ==
  in_bus : Inport
  Bus Selector : BusSelector  OutputSignals=AeroIn_Bus.angleOfAttack_deg,AeroIn_Bus.dAY,AeroIn_Bus.angleOfSideslip_deg,AeroIn_Bus.tflow,eoeff
  Ccdayb_ : Subsystem
  Ccdayb : Outport
  wires:
  Bus Selector/1 -> Ccdayb_/1(angleOfAttack_deg)  "<angleOfAttack_deg>"
  Bus Selector/2 -> Ccdayb_/2(dAY)  "<dAY>"
  Bus Selector/3 -> Ccdayb_/3(angleOfSideslip_deg)  "<angleOfSideslip_deg>"
  Bus Selector/4 -> Ccdayb_/4(tflow)  "<tflow>"
  Bus Selector/5 -> Ccdayb_/5(eoeff)  "<eoeff>"
  Ccdayb_/1(Ccdaib) -> Ccdayb/1
  in_bus/1 -> Bus Selector/1  "in_bus"

== system ADMIRE/Aircraft/Aerodynamics/CentripetalForceCoefficient/MachRegion2/Ccdna ==
  in_bus : Inport
  Bus Selector : BusSelector  OutputSignals=AeroIn_Bus.dNE,AeroIn_Bus.angleOfAttack_deg,AeroIn_Bus.tflow,AeroIn_Bus.tfhigh,AeroIn_Bus.dNA
  Ccdna_ : Subsystem
  Ccdna : Outport
  wires:
  Bus Selector/5 -> Ccdna_/5(dNA)  "<dNA>"
  Bus Selector/4 -> Ccdna_/4(tfhigh)  "<tfhigh>"
  Bus Selector/3 -> Ccdna_/3(tflow)  "<tflow>"
  Bus Selector/2 -> Ccdna_/2(angleOfAttack_deg)  "<angleOfAttack_deg>"
  Bus Selector/1 -> Ccdna_/1(dNE)  "<dNE>"
  in_bus/1 -> Bus Selector/1  "in_bus"
  Ccdna_/1(Ccdna) -> Ccdna/1

== system ADMIRE/Aircraft/Aerodynamics/CentripetalForceCoefficient/MachRegion2/Ccdr ==
  in_bus : Inport
  Bus Selector : BusSelector  OutputSignals=AeroIn_Bus.angleOfAttack_deg,AeroIn_Bus.rud_deg,AeroIn_Bus.angleOfSideslip_deg,AeroIn_Bus.tflow,AeroIn_Bus.tfhigh,AeroIn_Bus.qacorr,AeroIn_Bus.mach_nd
  Ccdr_ : Subsystem
  Ccdr : Outport
  wires:
  Bus Selector/7 -> Ccdr_/7(mach_nd)  "<mach_nd>"
  Bus Selector/6 -> Ccdr_/6(qacorr)  "<qacorr>"
  Bus Selector/5 -> Ccdr_/5(tfhigh)  "<tfhigh>"
  Bus Selector/4 -> Ccdr_/4(tflow)  "<tflow>"
  Bus Selector/3 -> Ccdr_/3(angleOfSideslip_deg)  "<angleOfSideslip_deg>"
  Bus Selector/2 -> Ccdr_/2(dR)  "<rud_deg>"
  Bus Selector/1 -> Ccdr_/1(angleOfAttack_deg)  "<angleOfAttack_deg>"
  Ccdr_/1(Ccdr) -> Ccdr/1
  in_bus/1 -> Bus Selector/1  "in_bus"

== system ADMIRE/Aircraft/Aerodynamics/CentripetalForceCoefficient/MachRegion2/Ccp ==
  in_bus : Inport
  Bus Selector : BusSelector  OutputSignals=AeroIn_Bus.angleOfAttack_deg,AeroIn_Bus.tflow,AeroIn_Bus.pc,AeroIn_Bus.tfhigh
  Ccp_ : Subsystem
  Ccp : Outport
  wires:
  Bus Selector/4 -> Ccp_/4(tfhigh)  "<tfhigh>"
  Bus Selector/3 -> Ccp_/3(pc)  "<pc>"
  Bus Selector/1 -> Ccp_/1(angleOfAttack_deg)  "<angleOfAttack_deg>"
  Bus Selector/2 -> Ccp_/2(tflow)  "<tflow>"
  in_bus/1 -> Bus Selector/1  "in_bus"
  Ccp_/1(Ccp) -> Ccp/1

== system ADMIRE/Aircraft/Aerodynamics/CentripetalForceCoefficient/MachRegion2/Ccpbeta ==
  in_bus : Inport
  Bus Selector : BusSelector  OutputSignals=AeroIn_Bus.angleOfSideslip_deg,AeroIn_Bus.angleOfAttack_deg,AeroIn_Bus.tflow,AeroIn_Bus.pc
  Ccpbeta_ : Subsystem
  Ccpbeta : Outport
  wires:
  Bus Selector/4 -> Ccpbeta_/4(pc)  "<pc>"
  Bus Selector/3 -> Ccpbeta_/3(tflow)  "<tflow>"
  Bus Selector/2 -> Ccpbeta_/2(angleOfAttack_deg)  "<angleOfAttack_deg>"
  Bus Selector/1 -> Ccpbeta_/1(angleOfSideslip_deg)  "<angleOfSideslip_deg>"
  Ccpbeta_/1(Ccpbeta) -> Ccpbeta/1
  in_bus/1 -> Bus Selector/1  "in_bus"

== system ADMIRE/Aircraft/Aerodynamics/CentripetalForceCoefficient/MachRegion2/Ccr ==
  in_bus : Inport
  Bus Selector : BusSelector  OutputSignals=AeroIn_Bus.dN,AeroIn_Bus.angleOfAttack_deg,AeroIn_Bus.tflow,AeroIn_Bus.tfhigh,AeroIn_Bus.rc,AeroIn_Bus.mach_nd,AeroIn_Bus.qacorr
  Ccr_ : Subsystem
  Ccr : Outport
  wires:
  Bus Selector/7 -> Ccr_/7(qacorr)  "<qacorr>"
  Bus Selector/6 -> Ccr_/6(mach_nd)  "<mach_nd>"
  Bus Selector/5 -> Ccr_/5(rc)  "<rc>"
  Bus Selector/4 -> Ccr_/4(tfhigh)  "<tfhigh>"
  Bus Selector/3 -> Ccr_/3(tflow)  "<tflow>"
  Bus Selector/2 -> Ccr_/2(angleOfAttack_deg)  "<angleOfAttack_deg>"
  Bus Selector/1 -> Ccr_/1(dN)  "<dN>"
  in_bus/1 -> Bus Selector/1  "in_bus"
  Ccr_/1(Ccr) -> Ccr/1

== system ADMIRE/Aircraft/Aerodynamics/CentripetalForceCoefficient/MachRegion2/Ccrbeta ==
  in_bus : Inport
  Bus Selector : BusSelector  OutputSignals=AeroIn_Bus.angleOfSideslip_deg,AeroIn_Bus.angleOfAttack_deg,AeroIn_Bus.tflow,AeroIn_Bus.rc
  Ccrbeta_ : Subsystem
  Ccrbeta : Outport
  wires:
  Bus Selector/1 -> Ccrbeta_/1(angleOfSideslip_deg)  "<angleOfSideslip_deg>"
  Bus Selector/2 -> Ccrbeta_/2(angleOfAttack_deg)  "<angleOfAttack_deg>"
  Bus Selector/4 -> Ccrbeta_/4(rc)  "<rc>"
  Bus Selector/3 -> Ccrbeta_/3(tflow)  "<tflow>"
  Ccrbeta_/1(Ccrbeta) -> Ccrbeta/1
  in_bus/1 -> Bus Selector/1  "in_bus"

== system ADMIRE/Aircraft/Aerodynamics/CentripetalForceCoefficient/MachRegion2/eoeff1 ==
  AeroIn_Bus : Inport
  Bus Selector : BusSelector  OutputSignals=mach_nd
  CCDAYOD_M : Lookup_n-D  NumberOfTableDimensions=1  BreakpointsForDimension1=admireDB.aerodata_asym_ext.CCDAYOD.breakpoints.M  BreakpointsForDimension3=[5, 7]  Table=admireDB.aerodata_asym_ext.CCDAYOD.newTable  ExtrapMethod=Clip  InternalRulePriority=Speed  RndMeth=Simplest  InputSameDT=on
  Constant : Constant
  Sum : Sum  Inputs=-+|
  eoeff : Outport
  eieff : Outport  Port=2
  wires:
  Sum/1 -> eieff/1
  CCDAYOD_M/1 -> eoeff/1, Sum/1
  Constant/1 -> Sum/2
  Bus Selector/1 -> CCDAYOD_M/1  "<mach_nd>"
  AeroIn_Bus/1 -> Bus Selector/1

== system ADMIRE/Aircraft/Aerodynamics/CentripetalForceCoefficient/MachRegion3/Ccbcai ==
  in_bus : Inport
  Bus Selector : BusSelector  OutputSignals=AeroIn_Bus.cai,AeroIn_Bus.angleOfAttack_deg,AeroIn_Bus.angleOfSideslip_deg
  Ccbcai_ : Subsystem
  Ccbcai : Outport
  wires:
  Bus Selector/1 -> Ccbcai_/1(cai)  "<cai>"
  Bus Selector/3 -> Ccbcai_/3(angleOfSideslip_deg)  "<angleOfSideslip_deg>"
  Bus Selector/2 -> Ccbcai_/2(angleOfAttack_deg)  "<angleOfAttack_deg>"
  in_bus/1 -> Bus Selector/1  "in_bus"
  Ccbcai_/1(Ccbcai) -> Ccbcai/1

== system ADMIRE/Aircraft/Aerodynamics/CentripetalForceCoefficient/MachRegion3/Ccbde ==
  in_bus : Inport
  Bus Selector : BusSelector  OutputSignals=AeroIn_Bus.angleOfAttack_deg,AeroIn_Bus.dEI,AeroIn_Bus.angleOfSideslip_deg,AeroIn_Bus.dEY,eieff,eoeff,AeroIn_Bus.mach_nd
  Ccbde_ : Subsystem
  Ccbde : Outport
  wires:
  Bus Selector/7 -> Ccbde_/7(mach_nd)  "<mach_nd>"
  Bus Selector/6 -> Ccbde_/6(eoeff)  "<eoeff>"
  Bus Selector/5 -> Ccbde_/5(eieff)  "<eieff>"
  Bus Selector/4 -> Ccbde_/4(dEY)  "<dEY>"
  Bus Selector/3 -> Ccbde_/3(angleOfSideslip_deg)  "<angleOfSideslip_deg>"
  Bus Selector/2 -> Ccbde_/2(dEI)  "<dEI>"
  Bus Selector/1 -> Ccbde_/1(angleOfAttack_deg)  "<angleOfAttack_deg>"
  Ccbde_/1(Ccbde) -> Ccbde/1
  in_bus/1 -> Bus Selector/1  "in_bus"

== system ADMIRE/Aircraft/Aerodynamics/CentripetalForceCoefficient/MachRegion3/Ccbdle ==
  in_bus : Inport
  Bus Selector : BusSelector  OutputSignals=AeroIn_Bus.mach_nd,AeroIn_Bus.angleOfAttack_deg,AeroIn_Bus.angleOfSideslip_deg,AeroIn_Bus.lef_deg
  Ccbdle_ : Subsystem
  Ccbdle : Outport
  wires:
  Bus Selector/4 -> Ccbdle_/4(dLE)  "<lef_deg>"
  Bus Selector/3 -> Ccbdle_/3(angleOfSideslip_deg)  "<angleOfSideslip_deg>"
  Bus Selector/1 -> Ccbdle_/1(mach_nd)  "<mach_nd>"
  Bus Selector/2 -> Ccbdle_/2(angleOfAttack_deg)  "<angleOfAttack_deg>"
  Ccbdle_/1(Ccbdle) -> Ccbdle/1
  in_bus/1 -> Bus Selector/1  "in_bus"

== system ADMIRE/Aircraft/Aerodynamics/CentripetalForceCoefficient/MachRegion3/Ccbdn ==
  in_bus : Inport
  Bus Selector : BusSelector  OutputSignals=AeroIn_Bus.angleOfAttack_deg,AeroIn_Bus.dN,AeroIn_Bus.angleOfSideslip_deg
  Ccbdn_ : Subsystem
  Ccbdn : Outport
  wires:
  Bus Selector/3 -> Ccbdn_/3(angleOfSideslip_deg)  "<angleOfSideslip_deg>"
  Bus Selector/2 -> Ccbdn_/2(dN)  "<dN>"
  Bus Selector/1 -> Ccbdn_/1(angleOfAttack_deg)  "<angleOfAttack_deg>"
  in_bus/1 -> Bus Selector/1  "in_bus"
  Ccbdn_/1(Ccbdn) -> Ccbdn/1

== system ADMIRE/Aircraft/Aerodynamics/CentripetalForceCoefficient/MachRegion3/Ccbeta ==
  in_bus : Inport
  Bus Selector : BusSelector  OutputSignals=AeroIn_Bus.mach_nd,AeroIn_Bus.angleOfAttack_deg,AeroIn_Bus.angleOfSideslip_deg,AeroIn_Bus.qacorr
  Ccbeta_ : Subsystem
  Ccbeta : Outport
  wires:
  Bus Selector/1 -> Ccbeta_/1(mach_nd)  "<mach_nd>"
  Bus Selector/2 -> Ccbeta_/2(angleOfAttack_deg)  "<angleOfAttack_deg>"
  Bus Selector/3 -> Ccbeta_/3(angleOfSideslip_deg)  "<angleOfSideslip_deg>"
  Bus Selector/4 -> Ccbeta_/4(qacorr)  "<qacorr>"
  Ccbeta_/1(CCbeta) -> Ccbeta/1
  in_bus/1 -> Bus Selector/1  "in_bus"

== system ADMIRE/Aircraft/Aerodynamics/CentripetalForceCoefficient/MachRegion3/Ccbetad ==
  in_bus : Inport
  Bus Selector : BusSelector  OutputSignals=AeroIn_Bus.angleOfAttack_deg,AeroIn_Bus.mach_nd,AeroIn_Bus.betad
  Ccbetad_ : Subsystem
  Ccbetad : Outport
  wires:
  Bus Selector/1 -> Ccbetad_/1(angleOfAttack_deg)  "<angleOfAttack_deg>"
  Bus Selector/2 -> Ccbetad_/2(mach_nd)  "<mach_nd>"
  Bus Selector/3 -> Ccbetad_/3(betad)  "<betad>"
  Ccbetad_/1(CCbetad) -> Ccbetad/1
  in_bus/1 -> Bus Selector/1  "in_bus"

== system ADMIRE/Aircraft/Aerodynamics/CentripetalForceCoefficient/MachRegion3/Ccblg ==
  in_bus : Inport
  Bus Selector : BusSelector  OutputSignals=AeroIn_Bus.lg_bool,AeroIn_Bus.angleOfAttack_deg,AeroIn_Bus.angleOfSideslip_deg
  Ccblg_ : Subsystem
  Ccblg : Outport
  wires:
  Bus Selector/1 -> Ccblg_/1(ldg)  "<lg_bool>"
  Bus Selector/3 -> Ccblg_/3(angleOfSideslip_deg)  "<angleOfSideslip_deg>"
  Bus Selector/2 -> Ccblg_/2(angleOfAttack_deg)  "<angleOfAttack_deg>"
  in_bus/1 -> Bus Selector/1  "in_bus"
  Ccblg_/1(Ccblg) -> Ccblg/1

== system ADMIRE/Aircraft/Aerodynamics/CentripetalForceCoefficient/MachRegion3/Ccdai ==
  in_bus : Inport
  Bus Selector : BusSelector  OutputSignals=AeroIn_Bus.angleOfAttack_deg,AeroIn_Bus.dAI,AeroIn_Bus.mach_nd,AeroIn_Bus.dEI,eieff,AeroIn_Bus.qacorr
  Ccdai_ : Subsystem
  Ccdai : Outport
  wires:
  Bus Selector/6 -> Ccdai_/6(qacorr)  "<qacorr>"
  Bus Selector/5 -> Ccdai_/5(eieff)  "<eieff>"
  Bus Selector/4 -> Ccdai_/4(dEI)  "<dEI>"
  Bus Selector/3 -> Ccdai_/3(mach_nd)  "<mach_nd>"
  Bus Selector/1 -> Ccdai_/1(angleOfAttack_deg)  "<angleOfAttack_deg>"
  Bus Selector/2 -> Ccdai_/2(dAI)  "<dAI>"
  in_bus/1 -> Bus Selector/1  "in_bus"
  Ccdai_/1(Ccdai) -> Ccdai/1

== system ADMIRE/Aircraft/Aerodynamics/CentripetalForceCoefficient/MachRegion3/Ccdaib ==
  Constant : Constant  Value=0
  Ccdaib : Outport
  wires:
  Constant/1 -> Ccdaib/1

== system ADMIRE/Aircraft/Aerodynamics/CentripetalForceCoefficient/MachRegion3/Ccday ==
  in_bus : Inport
  Bus Selector : BusSelector  OutputSignals=AeroIn_Bus.angleOfAttack_deg,AeroIn_Bus.dAY,AeroIn_Bus.mach_nd,AeroIn_Bus.dEY,eoeff,AeroIn_Bus.qacorr
  Ccday_ : Subsystem
  Ccday : Outport
  wires:
  Ccday_/1(Ccday) -> Ccday/1
  in_bus/1 -> Bus Selector/1  "in_bus"
  Bus Selector/2 -> Ccday_/2(dAY)  "<dAY>"
  Bus Selector/1 -> Ccday_/1(angleOfAttack_deg)  "<angleOfAttack_deg>"
  Bus Selector/3 -> Ccday_/3(mach_nd)  "<mach_nd>"
  Bus Selector/4 -> Ccday_/4(dEY)  "<dEY>"
  Bus Selector/5 -> Ccday_/5(eoeff)  "<eoeff>"
  Bus Selector/6 -> Ccday_/6(qacorr)  "<qacorr>"

== system ADMIRE/Aircraft/Aerodynamics/CentripetalForceCoefficient/MachRegion3/Ccdayb ==
  Constant : Constant  Value=0
  Ccdayb : Outport
  wires:
  Constant/1 -> Ccdayb/1

== system ADMIRE/Aircraft/Aerodynamics/CentripetalForceCoefficient/MachRegion3/Ccdna ==
  in_bus : Inport
  Bus Selector : BusSelector  OutputSignals=AeroIn_Bus.angleOfAttack_deg,AeroIn_Bus.mach_nd,AeroIn_Bus.dNA
  Ccdna_ : Subsystem
  Ccdna : Outport
  wires:
  Bus Selector/1 -> Ccdna_/1(angleOfAttack_deg)  "<angleOfAttack_deg>"
  Bus Selector/3 -> Ccdna_/3(dNA)  "<dNA>"
  Bus Selector/2 -> Ccdna_/2(mach_nd)  "<mach_nd>"
  in_bus/1 -> Bus Selector/1  "in_bus"
  Ccdna_/1(Ccdna) -> Ccdna/1

== system ADMIRE/Aircraft/Aerodynamics/CentripetalForceCoefficient/MachRegion3/Ccdr ==
  in_bus : Inport
  Bus Selector : BusSelector  OutputSignals=AeroIn_Bus.angleOfAttack_deg,AeroIn_Bus.mach_nd,AeroIn_Bus.rud_deg,AeroIn_Bus.qacorr
  Ccdr_ : Subsystem
  Ccdr : Outport
  wires:
  Bus Selector/1 -> Ccdr_/1(angleOfAttack_deg)  "<angleOfAttack_deg>"
  Bus Selector/2 -> Ccdr_/2(mach_nd)  "<mach_nd>"
  Bus Selector/3 -> Ccdr_/3(dR)  "<rud_deg>"
  Bus Selector/4 -> Ccdr_/4(qacorr)  "<qacorr>"
  Ccdr_/1(Ccdr) -> Ccdr/1
  in_bus/1 -> Bus Selector/1  "in_bus"

== system ADMIRE/Aircraft/Aerodynamics/CentripetalForceCoefficient/MachRegion3/Ccp1 ==
  in_bus : Inport
  Bus Selector : BusSelector  OutputSignals=AeroIn_Bus.angleOfAttack_deg,AeroIn_Bus.mach_nd,AeroIn_Bus.pc
  Ccp_ : Subsystem
  Ccp : Outport
  wires:
  Bus Selector/1 -> Ccp_/1(angleOfAttack_deg)  "<angleOfAttack_deg>"
  Bus Selector/2 -> Ccp_/2(mach_nd)  "<mach_nd>"
  Bus Selector/3 -> Ccp_/3(pc)  "<pc>"
  in_bus/1 -> Bus Selector/1  "in_bus"
  Ccp_/1(Ccp) -> Ccp/1

== system ADMIRE/Aircraft/Aerodynamics/CentripetalForceCoefficient/MachRegion3/Ccpbeta ==
  Constant : Constant  Value=0
  Ccpbeta : Outport
  wires:
  Constant/1 -> Ccpbeta/1

== system ADMIRE/Aircraft/Aerodynamics/CentripetalForceCoefficient/MachRegion3/Ccr1 ==
  in_bus : Inport
  Bus Selector : BusSelector  OutputSignals=AeroIn_Bus.mach_nd,AeroIn_Bus.rc
  Ccr_ : Subsystem
  Ccr : Outport
  wires:
  Bus Selector/2 -> Ccr_/2(rc)  "<rc>"
  Bus Selector/1 -> Ccr_/1(mach_nd)  "<mach_nd>"
  in_bus/1 -> Bus Selector/1  "in_bus"
  Ccr_/1(Ccr) -> Ccr/1

== system ADMIRE/Aircraft/Aerodynamics/CentripetalForceCoefficient/MachRegion3/Ccrbeta ==
  Constant : Constant  Value=0
  Ccrbeta : Outport
  wires:
  Constant/1 -> Ccrbeta/1

== system ADMIRE/Aircraft/Aerodynamics/CentripetalForceCoefficient/MachRegion3/eoeff1 ==
  AeroIn_Bus : Inport
  Bus Selector : BusSelector  OutputSignals=mach_nd
  CCDAYOD_M : Lookup_n-D  NumberOfTableDimensions=1  BreakpointsForDimension1=admireDB.aerodata_asym_ext.CCDAYOD.breakpoints.M  BreakpointsForDimension3=[5, 7]  Table=admireDB.aerodata_asym_ext.CCDAYOD.newTable  ExtrapMethod=Clip  InternalRulePriority=Speed  RndMeth=Simplest  InputSameDT=on
  Constant : Constant
  Sum : Sum  Inputs=-+|
  eoeff : Outport
  eieff : Outport  Port=2
  wires:
  Sum/1 -> eieff/1
  CCDAYOD_M/1 -> eoeff/1, Sum/1
  Constant/1 -> Sum/2
  Bus Selector/1 -> CCDAYOD_M/1  "<mach_nd>"
  AeroIn_Bus/1 -> Bus Selector/1

== system ADMIRE/Aircraft/Aerodynamics/CentripetalForceCoefficient/MachRegion4/Ccbcai ==
  in_bus : Inport
  Bus Selector : BusSelector  OutputSignals=AeroIn_Bus.cai,AeroIn_Bus.angleOfAttack_deg,AeroIn_Bus.angleOfSideslip_deg
  Ccbcai_ : Subsystem
  Ccbcai : Outport
  wires:
  Bus Selector/1 -> Ccbcai_/1(cai)  "<cai>"
  Bus Selector/3 -> Ccbcai_/3(angleOfSideslip_deg)  "<angleOfSideslip_deg>"
  Bus Selector/2 -> Ccbcai_/2(angleOfAttack_deg)  "<angleOfAttack_deg>"
  in_bus/1 -> Bus Selector/1  "in_bus"
  Ccbcai_/1(Ccbcai) -> Ccbcai/1

== system ADMIRE/Aircraft/Aerodynamics/CentripetalForceCoefficient/MachRegion4/Ccbde ==
  in_bus : Inport
  Bus Selector : BusSelector  OutputSignals=AeroIn_Bus.angleOfAttack_deg,AeroIn_Bus.dEI,AeroIn_Bus.angleOfSideslip_deg,AeroIn_Bus.dEY,eieff,eoeff,AeroIn_Bus.mach_nd
  Ccbde_ : Subsystem
  Ccbde : Outport
  wires:
  Bus Selector/7 -> Ccbde_/7(mach_nd)  "<mach_nd>"
  Bus Selector/6 -> Ccbde_/6(eoeff)  "<eoeff>"
  Bus Selector/5 -> Ccbde_/5(eieff)  "<eieff>"
  Bus Selector/4 -> Ccbde_/4(dEY)  "<dEY>"
  Bus Selector/3 -> Ccbde_/3(angleOfSideslip_deg)  "<angleOfSideslip_deg>"
  Bus Selector/2 -> Ccbde_/2(dEI)  "<dEI>"
  Bus Selector/1 -> Ccbde_/1(angleOfAttack_deg)  "<angleOfAttack_deg>"
  Ccbde_/1(Ccbde) -> Ccbde/1
  in_bus/1 -> Bus Selector/1  "in_bus"
